simulink model "WaterTank"  (Simulink 6.5)
settings: Solver=ode45  StartTime=0.0  StopTime=1000  RelTol=1e-3
InitFcn:
  | g = 9.81; %gravitational constant
  | 
  | %% S-function
  | % showVR = 0;
  | % h0 = 0; %initial conditions
libraries: vrlib x5
CloseFcn:
  | vrclose all;
  | clear figureVR worldVR;
settings Model: Creator=Owner  LastModifiedBy=Jirka

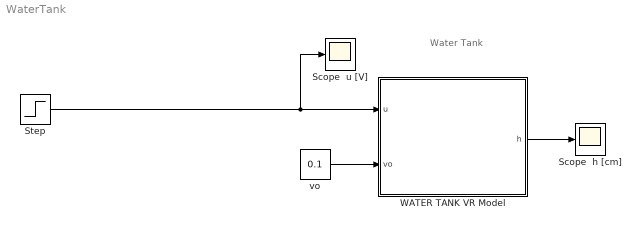
== system WaterTank ==
  note: Water Tank
  Scope  h [cm] : Scope
      settings: TimeRange=1000  YMin=0  YMax=25  SaveName=ty  DataFormat=Array  MaxDataPoints=50000
  Scope  u [V] : Scope
      settings: TimeRange=1000  YMin=-2  YMax=12  SaveName=tu  DataFormat=Array  MaxDataPoints=50000
  Step : Step  Time=400  Before=7  After=5  SampleTime=0
  WATER TANK VR Model : Subsystem  mask(Water tank){showVR=on, sfcnParam1=0}
      mask prompts: showVR "Show VirtualWorld?"; sfcnParam1 "Initial fluid level in the tank   h(0) [cm]"
      mask help: WaterTank - Virtual Reality
      mask init:
      | clear figureVR worldVR;
      | showVR = 1;
      mask Help:
      | WaterTank - Virtual Reality. <br><br>
      | 
      | 
      | This is a model of the water tank, which consists of a gear-pump, tank, inflow and outflow pipes and  output valve.
      | The tank is filled with the fluid by the gear-pump and the fluid drains away through the output valve. The system
      | inputs are the voltage of the motor of the gear-pump and the output valve opening. The system output is the level
      | of the fluid in the tank. The dynamics of the gear-pump is neglected. <br><br>
      | 
      | 
      | In the mask of the model, it can be set:
      | <ul>
      | <li>Initial fluid level in the tank.</li>
      | </ul><br><br>
      | 
      | 
      | Copyright: 2007,   Jan Vana, Jirka Roubal, Petr Husek.
      mask CallbackString:
      | if strcmp('off',get_param(gcb,'showVR'))
      |     vrclose all;
      | else
      |     if exist('figureVR')==0
      |         figureVR = vrfigure;
      |     end
      |     if exist('worldVR')==0
      |         worldVR = vrworld('WaterTank_VR.WRL');
      |     end
      | 	if isvalid(figureVR)==0
      |         open(worldVR);
      |         figureVR = vrfigure(worldVR,[650 80 550 350]);
      | 	end
      | end|
      mask Display:
      | image(imread('WaterTank_Image.jpg'))
      | port_label ('input',1,'u')
      | port_label ('input',2,'vo')
      | port_label ('output',1,'h')
  vo : Constant  Value=0.1  OutDataType=sfix(16)  ConRadixGroup=Use specified scaling  OutScaling=2^0  SampleTime=inf  FramePeriod=inf
  wires:
  Step/1 -> Scope  u [V]/1, WATER TANK VR Model/1(u)
  WATER TANK VR Model/1(h) -> Scope  h [cm]/1
  vo/1 -> WATER TANK VR Model/2(vo)

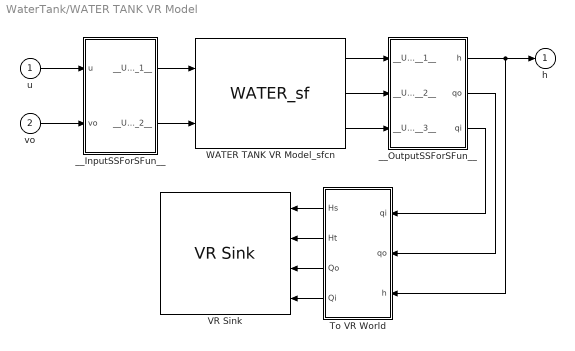
== system WaterTank/WATER TANK VR Model ==
  u : Inport
  vo : Inport  Port=2
  To VR World : Subsystem  Orientation=left
  VR Sink : vrlib/VR Sink  Orientation=left  SampleTime=0.1  ViewEnable=on  RemoteChange=off  RemoteView=on  FieldsWritten=water.scale.3.1.double#water.translation.3.1.double#pumpOut.rotation.4.1.double#pumpIn.rotation.4.1.double  WorldFileName=WaterTank_VR.wrl  AutoView=off  FigureProperties={}
  WATER TANK VR Model_sfcn : S-Function  FunctionName=WATER_sf  Parameters=sfcnParam1  SFunctionModules=""  mask{rtw_sf_name=WATER_sf, showVar=off, sfcnParam1=sfcnParam1}
      mask prompts: rtw_sf_name "Generated S-function name (model_sf):"; showVar "Show module list"; sfcnParam1 "h0:"
      mask help: Real-Time Workshop generated S-function.
      mask init:
      | displist = '';
      | if ~strcmp(get_param(gcb, 'FunctionName'), rtw_sf_name);
      |   set_param(gcb, 'FunctionName', rtw_sf_name);
      | end
      | % Check if we are generating RTW code
      | rtw_mode = false;
      | if strcmpi(get_param(bdroot(gcb),'SimulationStatus'),'Initializing')
      | 	rtw_mode = strcmpi(get_param(bdroot(gcb),'BuildingRTWCode'),'on') && ...
      | 		~strcmpi(get_param(bdroot(gcb),'TargetStyle'),'SimulationTarget');
      | end
      | if showVar || rtw_mode
      | 	if exist('rtwsfunc') == 2 | exist('rtwsfunc') == 6
      | 		tmplist = rtwsfunc(rtw_sf_name,gcb);
      | 		tmplist = ['\nList of Modules:\n', tmplist];
      | 	elseif showVar
      | 		tmplist = '\nList of Modules:\nRTW not licensed\n';
      |  	end
      | end
      | if showVar
      |   displist = tmplist;
      | end
      settings: CopyFcn=set_param(gcb,'LinkStatus','none');
      mask Help: helpview([docroot,'\toolbox\rtw\helptargets.map'],'rtw_Sfunc_target');
      mask Display:
      | port_label('input',1,'u');
      | port_label('input',2,'vo');
      | port_label('output',1,'h');
      | port_label('output',2,'qo');
      | port_label('output',3,'qi');
  __InputSSForSFun__ : Subsystem
  __OutputSSForSFun__ : Subsystem
  h : Outport  PortDimensions=1  SampleTime=[-1 0]  DataType=double
  wires:
  __OutputSSForSFun__/2(qo) -> To VR World/2(qo)
  __OutputSSForSFun__/3(qi) -> To VR World/1(qi)
  To VR World/4(Qi) -> VR Sink/4
  To VR World/3(Qo) -> VR Sink/3
  To VR World/2(Ht) -> VR Sink/2
  To VR World/1(Hs) -> VR Sink/1
  __OutputSSForSFun__/1(h) -> h/1, To VR World/3(h)
  WATER TANK VR Model_sfcn/3 -> __OutputSSForSFun__/3(__UniqueInportName__3__)
  WATER TANK VR Model_sfcn/2 -> __OutputSSForSFun__/2(__UniqueInportName__2__)
  WATER TANK VR Model_sfcn/1 -> __OutputSSForSFun__/1(__UniqueInportName__1__)
  __InputSSForSFun__/2(__UniqueOutportName__2__) -> WATER TANK VR Model_sfcn/2
  __InputSSForSFun__/1(__UniqueOutportName__1__) -> WATER TANK VR Model_sfcn/1
  vo/1 -> __InputSSForSFun__/2(vo)
  u/1 -> __InputSSForSFun__/1(u)

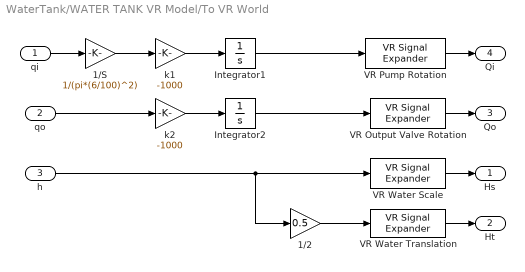
== system WaterTank/WATER TANK VR Model/To VR World ==
  qi : Inport
  qo : Inport  Port=2
  h : Inport  Port=3
  1/2 : Gain  Gain=0.5
  1/S : Gain  Gain=1/(pi*(6/100)^2)
  Integrator1 : Integrator
  Integrator2 : Integrator
  VR Output Valve Rotation : vrlib/VR Signal Expander  SystemSampleTime=-1  outwidth=4  outidx=[4]
  VR Pump Rotation : vrlib/VR Signal Expander  SystemSampleTime=-1  outwidth=4  outidx=[4]
  VR Water Scale : vrlib/VR Signal Expander  SystemSampleTime=-1  outwidth=3  outidx=[2]
  VR Water Translation : vrlib/VR Signal Expander  SystemSampleTime=-1  outwidth=3  outidx=[2]
  k1 : Gain  Gain=-1000
  k2 : Gain  Gain=-1000
  Hs : Outport
  Ht : Outport  Port=2
  Qo : Outport  Port=3
  Qi : Outport  Port=4
  wires:
  1/2/1 -> VR Water Translation/1
  Integrator2/1 -> VR Output Valve Rotation/1
  Integrator1/1 -> VR Pump Rotation/1
  qi/1 -> 1/S/1
  qo/1 -> k2/1
  h/1 -> 1/2/1, VR Water Scale/1
  VR Pump Rotation/1 -> Qi/1
  VR Output Valve Rotation/1 -> Qo/1
  VR Water Scale/1 -> Hs/1
  VR Water Translation/1 -> Ht/1
  k2/1 -> Integrator2/1
  k1/1 -> Integrator1/1
  1/S/1 -> k1/1

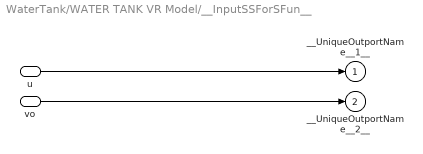
== system WaterTank/WATER TANK VR Model/__InputSSForSFun__ ==
  u : Inport
  vo : Inport  Port=2
  __UniqueOutportName__1__ : Outport
  __UniqueOutportName__2__ : Outport  Port=2
  wires:
  vo/1 -> __UniqueOutportName__2__/1
  u/1 -> __UniqueOutportName__1__/1

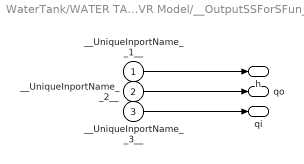
== system WaterTank/WATER TANK VR Model/__OutputSSForSFun__ ==
  __UniqueInportName__1__ : Inport
  __UniqueInportName__2__ : Inport  Port=2
  __UniqueInportName__3__ : Inport  Port=3
  h : Outport  PortDimensions=1  SampleTime=[-1 0]  DataType=double
  qo : Outport  Port=2  PortDimensions=1  SampleTime=[-1 0]  DataType=double
  qi : Outport  Port=3  PortDimensions=1  SampleTime=[0 1]  DataType=double
  wires:
  __UniqueInportName__3__/1 -> qi/1
  __UniqueInportName__2__/1 -> qo/1
  __UniqueInportName__1__/1 -> h/1
